simulink model "DSM1"  (R2020a)
settings: Solver=VariableStepAuto  StartTime=0.0  StopTime=0.6  RelTol=1e-3
settings Model: Creator=bzhan  LastModifiedBy=bzhan

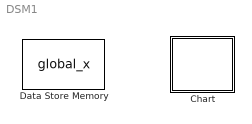
== system DSM1 ==
  Chart : Stateflow chart  TreatAsAtomicUnit=on
  Data Store Memory : DataStoreMemory  DataStoreName=global_x  ReadBeforeWriteMsg=warning  WriteAfterWriteMsg=warning  WriteAfterReadMsg=warning  ShowAdditionalParam=off  OutDataTypeStr=int32

== stateflow chart DSM1/Chart ==
  settings: updateMethod=DISCRETE  sampleTime=0.1
  state A
  state B
  (default) -> A : {global_x = 1;}
  A -> B : {global_x = global_x + 1;f()}
  B -> A : {global_x = global_x + 2;f()}
  data: global_x data_store_memory
  function f:
    | function f
    |   fprintf("%d\n", global_x);
